simulink library "TorqueVectoringAlgorithmLib"  (R2020a)
settings: Solver=VariableStepAuto  StartTime=0.0  StopTime=10.0  RelTol=1e-3
undefined symbols (not defined in the file): VDR
settings Model: Creator=Harjot  LastModifiedBy=Harjot
settings DebuggingCC: ArithmeticOperatorsInVariantConditions=warning
settings SFSimCC: SimUseLocalCustomCode=off  CustomCodeUndefinedFunction=UseInterfaceOnly
settings RTWCC: RTWUseLocalCustomCode=off

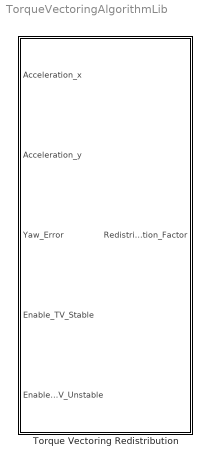
== system TorqueVectoringAlgorithmLib ==
  Torque Vectoring Redistribution : Subsystem  mask{wheel_1=Front, wheel_2=Left}
      mask prompts: wheel_1 "Front or Rear Wheel"; wheel_2 "Left or Right Wheel"
      mask init:
      | %Front vs Rear Modifier
      | if(wheel_1 == 1) %Front Wheel
      |     stable_longitudinal_mod = -1;
      | else %Rear Wheel
      |     stable_longitudinal_mod = 1;
      | end
      | 
      | %Left vs Rear Modifier
      | if(wheel_2 == 1) %Left Wheel
      |     unstable_mod = -1;
      |     stable_lateral_mod = -1;
      | else %Right Wheel
      |     unstable_mod = 1;
      |     stable_lateral_mod = 1;
      | end
      mask TypeOptions wheel_1: Front | Rear
      mask TypeOptions wheel_2: Left | Right
      mask DialogControl DescGroupVar Prompt: Torque Vectoring Configurations
      mask DialogControl DescTextVar Prompt: Select the wheel for the torque vectoring configuration.

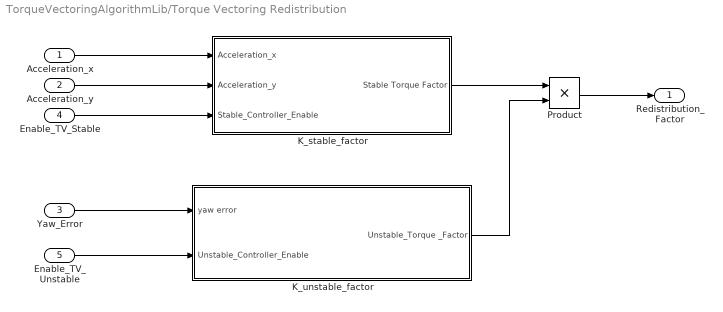
== system TorqueVectoringAlgorithmLib/Torque Vectoring Redistribution ==
  Acceleration_x : Inport
  Acceleration_y : Inport  Port=2
  Yaw_Error : Inport  Port=3
  Enable_TV_Stable : Inport  Port=4
  Enable_TV_Unstable : Inport  Port=5
  K_stable_factor : Subsystem
  K_unstable_factor : Subsystem
  Product : Product
  Redistribution_Factor : Outport  VectorParamsAs1DForOutWhenUnconnected=off
  wires:
  K_unstable_factor/1(Unstable_Torque _Factor) -> Product/2
  K_stable_factor/1(Stable Torque Factor) -> Product/1
  Acceleration_x/1 -> K_stable_factor/1(Acceleration_x)
  Yaw_Error/1 -> K_unstable_factor/1(yaw error)
  Acceleration_y/1 -> K_stable_factor/2(Acceleration_y)
  Product/1 -> Redistribution_Factor/1
  Enable_TV_Stable/1 -> K_stable_factor/3(Stable_Controller_Enable)
  Enable_TV_Unstable/1 -> K_unstable_factor/2(Unstable_Controller_Enable)

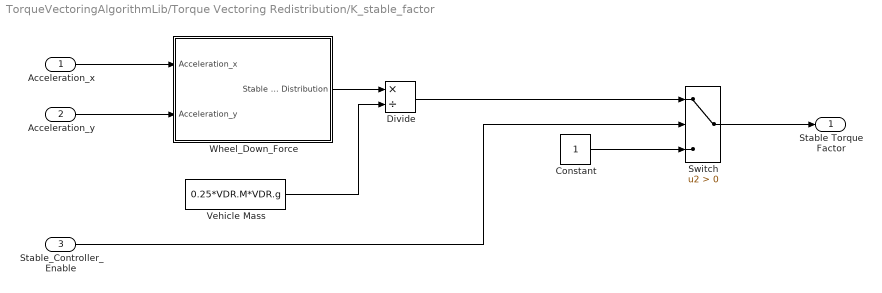
== system TorqueVectoringAlgorithmLib/Torque Vectoring Redistribution/K_stable_factor ==
  Acceleration_x : Inport
  Acceleration_y : Inport  Port=2
  Stable_Controller_Enable : Inport  Port=3
  Constant : Constant
  Divide : Product  Inputs=*/
  Switch : Switch  Criteria=u2 > Threshold
  Vehicle Mass : Constant  Value=0.25*VDR.M*VDR.g
  Wheel_Down_Force : Subsystem
  Stable Torque Factor : Outport  VectorParamsAs1DForOutWhenUnconnected=off
  wires:
  Acceleration_y/1 -> Wheel_Down_Force/2(Acceleration_y)
  Acceleration_x/1 -> Wheel_Down_Force/1(Acceleration_x)
  Wheel_Down_Force/1(Stable Weigth Distribution) -> Divide/1
  Vehicle Mass/1 -> Divide/2
  Stable_Controller_Enable/1 -> Switch/2
  Divide/1 -> Switch/1
  Switch/1 -> Stable Torque Factor/1
  Constant/1 -> Switch/3

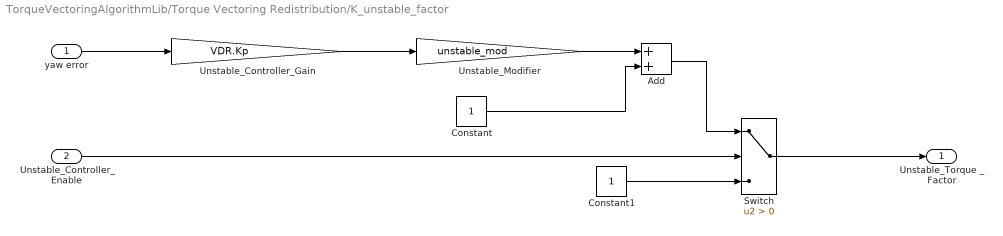
== system TorqueVectoringAlgorithmLib/Torque Vectoring Redistribution/K_unstable_factor ==
  yaw error : Inport
  Unstable_Controller_Enable : Inport  Port=2
  Add : Sum
  Constant : Constant
  Constant1 : Constant
  Switch : Switch  Criteria=u2 > Threshold
  Unstable_Controller_Gain : Gain  Gain=VDR.Kp
  Unstable_Modifier : Gain  Gain=unstable_mod
  Unstable_Torque _Factor : Outport  VectorParamsAs1DForOutWhenUnconnected=off
  wires:
  Unstable_Controller_Gain/1 -> Unstable_Modifier/1
  Constant/1 -> Add/2
  yaw error/1 -> Unstable_Controller_Gain/1
  Unstable_Modifier/1 -> Add/1
  Add/1 -> Switch/1
  Switch/1 -> Unstable_Torque _Factor/1
  Unstable_Controller_Enable/1 -> Switch/2
  Constant1/1 -> Switch/3

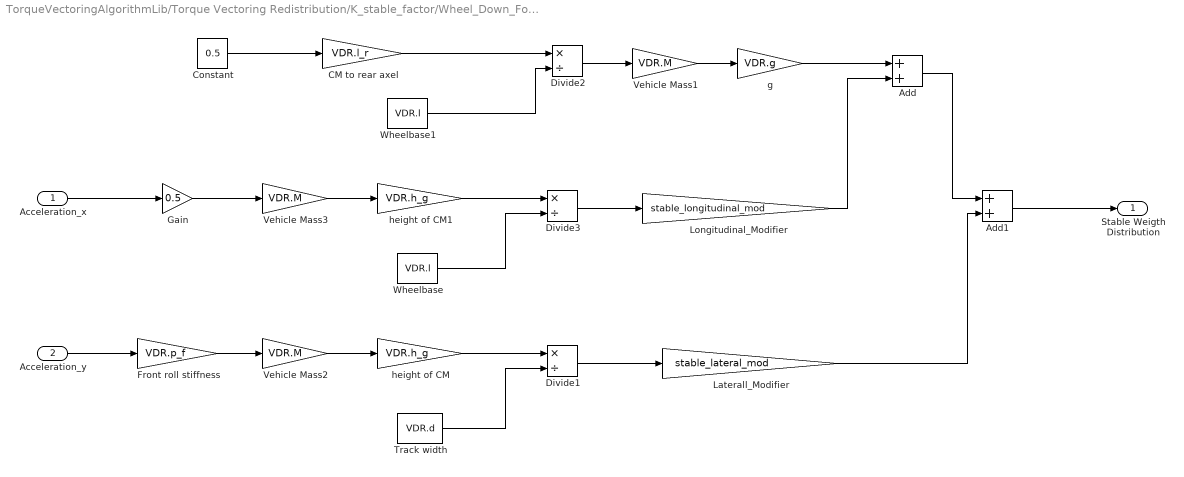
== system TorqueVectoringAlgorithmLib/Torque Vectoring Redistribution/K_stable_factor/Wheel_Down_Force ==
  Acceleration_x : Inport
  Acceleration_y : Inport  Port=2
  Add : Sum
  Add1 : Sum
  CM to rear axel : Gain  Gain=VDR.l_r
  Constant : Constant  Value=0.5
  Divide1 : Product  Inputs=*/
  Divide2 : Product  Inputs=*/
  Divide3 : Product  Inputs=*/
  Front roll stiffness : Gain  Gain=VDR.p_f
  Gain : Gain  Gain=0.5
  Laterall_Modifier : Gain  Gain=stable_lateral_mod
  Longitudinal_Modifier : Gain  Gain=stable_longitudinal_mod
  Track width : Constant  Value=VDR.d
  Vehicle Mass1 : Gain  Gain=VDR.M
  Vehicle Mass2 : Gain  Gain=VDR.M
  Vehicle Mass3 : Gain  Gain=VDR.M
  Wheelbase : Constant  Value=VDR.l
  Wheelbase1 : Constant  Value=VDR.l
  g : Gain  Gain=VDR.g
  height of CM : Gain  Gain=VDR.h_g
  height of CM1 : Gain  Gain=VDR.h_g
  Stable Weigth Distribution : Outport  VectorParamsAs1DForOutWhenUnconnected=off
  wires:
  Add1/1 -> Stable Weigth Distribution/1
  height of CM1/1 -> Divide3/1
  Vehicle Mass3/1 -> height of CM1/1
  height of CM/1 -> Divide1/1
  Vehicle Mass2/1 -> height of CM/1
  Vehicle Mass1/1 -> g/1
  Front roll stiffness/1 -> Vehicle Mass2/1
  Acceleration_x/1 -> Gain/1
  CM to rear axel/1 -> Divide2/1
  Constant/1 -> CM to rear axel/1
  Acceleration_y/1 -> Front roll stiffness/1
  Divide2/1 -> Vehicle Mass1/1
  Wheelbase1/1 -> Divide2/2
  Divide3/1 -> Longitudinal_Modifier/1
  Divide1/1 -> Laterall_Modifier/1
  Wheelbase/1 -> Divide3/2
  Track width/1 -> Divide1/2
  g/1 -> Add/1
  Longitudinal_Modifier/1 -> Add/2
  Add/1 -> Add1/1
  Laterall_Modifier/1 -> Add1/2
  Gain/1 -> Vehicle Mass3/1
